simulink model "BIKENON"  (R2023a)
settings: Solver=ode113  StartTime=0.0  StopTime=15  MaxStep=1  RelTol=1e-3  AbsTol=1e-3
values from neighbouring files (symbols this model uses):
  u0 = initial_velocities(v_idx)    [perform_simulations.m]    (also in plots.m = initialVelocities(vIdx))
undefined symbols (not defined in the file or in its folder): a, b, Cf, Cr, G, I, M, r0, v0
settings Model: Creator=pisup  LastModifiedBy=kvadner
settings SolverCC: AutoScaleAbsTol=off  AlgebraicLoopSolver=TrustRegion
settings DataIOCC: SaveFormat=Array  SignalLoggingSaveFormat=ModelDataLogs  SaveOutput=off  SaveTime=off  ReturnWorkspaceOutputs=off
settings OptimizationCC: BlockReduction=off  BooleanDataType=off  ExpressionDepthLimit=2147483647  InitFltsAndDblsToZero=on  LifeSpan=inf
settings DebuggingCC: SaveWithParameterizedLinksMsg=none  UnderspecifiedInitializationDetection=Classic  MergeDetectMultiDrivingBlocksExec=none  SignalResolutionControl=TryResolveAllWithWarning  MultiTaskDSMMsg=warning  MultiTaskCondExecSysMsg=none  FcnCallInpInsideContextMsg=warning  UnconnectedInputMsg=warning  UnconnectedOutputMsg=warning  UnconnectedLineMsg=warning  StateNameClashWarn=warning  SFUnexpectedBacktrackingDiag=warning  SFNoUnconditionalDefaultTransitionDiag=warning  SFExecutionAtInitializationDiag=none  ArithmeticOperatorsInVariantConditions=warning
settings HardwareCC: ProdBitPerPointer=32  ProdBitPerSizeT=32  ProdBitPerPtrDiffT=32  ProdLargestAtomicFloat=None  ProdIntDivRoundTo=Undefined  ProdEndianess=Unspecified  ProdWordSize=32  ProdHWDeviceType=32-bit Generic  TargetUnknown=on
settings ModelReferenceCC: EnableRefExpFcnMdlSchedulingChecks=on  PropagateSignalLabelsOutOfModel=off
settings RTWCC: TemplateMakefile=grt_vc.tmf
settings CodeAppCC: StateflowObjectComments=on
settings GRTTargetCC: TargetLangStandard=C89/C90 (ANSI)  CombineOutputUpdateFcns=off  GRTInterface=on
settings ConfigComp: CovMetricSettings=dw  CovSaveCumulativeToWorkspaceVar=on  CovSaveSingleToWorkspaceVar=on

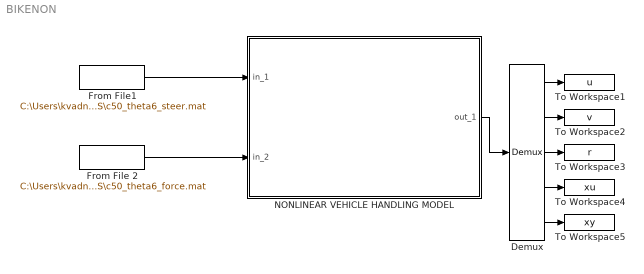
== system BIKENON ==
  Demux : Demux  Outputs=5
      settings: DisplayOption=none
  From File 2 : FromFile  FileName=C:\Users\kvadner\Desktop\Research\Fault Detection Markov MDP\Simulink\Files for HW2\Input Maneuvers\SRS\c50_theta6_force.mat  SampleTime=0
  From File1 : FromFile  FileName=C:\Users\kvadner\Desktop\Research\Fault Detection Markov MDP\Simulink\Files for HW2\Input Maneuvers\SRS\c50_theta6_steer.mat  SampleTime=0
  NONLINEAR VEHICLE HANDLING MODEL : Subsystem
  To Workspace1 : ToWorkspace  VariableName=u
      settings: MaxDataPoints=10000
  To Workspace2 : ToWorkspace  VariableName=v
      settings: MaxDataPoints=10000
  To Workspace3 : ToWorkspace  VariableName=r
      settings: MaxDataPoints=10000
  To Workspace4 : ToWorkspace  VariableName=xu
      settings: MaxDataPoints=10000
  To Workspace5 : ToWorkspace  VariableName=xy
      settings: MaxDataPoints=10000
  wires:
  Demux/3 -> To Workspace3/1
  Demux/2 -> To Workspace2/1
  Demux/1 -> To Workspace1/1
  NONLINEAR VEHICLE HANDLING MODEL/1(out_1) -> Demux/1
  Demux/4 -> To Workspace4/1
  Demux/5 -> To Workspace5/1
  From File1/1 -> NONLINEAR VEHICLE HANDLING MODEL/1(in_1)
  From File 2/1 -> NONLINEAR VEHICLE HANDLING MODEL/2(in_2)

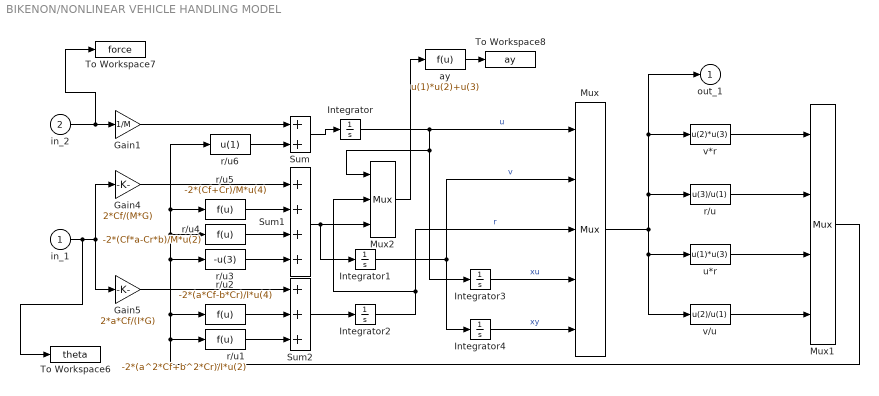
== system BIKENON/NONLINEAR VEHICLE HANDLING MODEL ==
  in_1 : Inport
  in_2 : Inport  Port=2
  Gain1 : Gain  Gain=1/M  SaturateOnIntegerOverflow=on  OutDataTypeStr=Inherit: Same as input  ParamDataTypeStr=Inherit: Same as input
  Gain4 : Gain  Gain=2*Cf/(M*G)  SaturateOnIntegerOverflow=on  OutDataTypeStr=Inherit: Same as input  ParamDataTypeStr=Inherit: Same as input
  Gain5 : Gain  Gain=2*a*Cf/(I*G)  SaturateOnIntegerOverflow=on  OutDataTypeStr=Inherit: Same as input  ParamDataTypeStr=Inherit: Same as input
  Integrator : Integrator  InitialCondition=u0
  Integrator1 : Integrator  InitialCondition=v0
  Integrator2 : Integrator  InitialCondition=r0
  Integrator3 : Integrator
  Integrator4 : Integrator
  Mux : Mux  Inputs=5
  Mux1 : Mux
  Mux2 : Mux  Inputs=3
  Sum : Sum  InputSameDT=on  SaturateOnIntegerOverflow=on  OutDataTypeStr=Inherit: Same as first input
  Sum1 : Sum  Inputs=++++  InputSameDT=on  SaturateOnIntegerOverflow=on  OutDataTypeStr=Inherit: Same as first input
  Sum2 : Sum  Inputs=+++  InputSameDT=on  SaturateOnIntegerOverflow=on  OutDataTypeStr=Inherit: Same as first input
  To Workspace6 : ToWorkspace  VariableName=theta
      settings: MaxDataPoints=10000
  To Workspace7 : ToWorkspace  VariableName=force
      settings: MaxDataPoints=10000
  To Workspace8 : ToWorkspace  VariableName=ay
      settings: MaxDataPoints=10000
  ay : Fcn  Expr=u(1)*u(2)+u(3)
  r/u : Fcn  Expr=u(3)/u(1)
  r/u1 : Fcn  Expr=-2*(a^2*Cf+b^2*Cr)/I*u(2)
  r/u2 : Fcn  Expr=-2*(a*Cf-b*Cr)/I*u(4)
  r/u3 : Fcn  Expr=-u(3)
  r/u4 : Fcn  Expr=-2*(Cf*a-Cr*b)/M*u(2)
  r/u5 : Fcn  Expr=-2*(Cf+Cr)/M*u(4)
  r/u6 : Fcn  Expr=u(1)
  u*r : Fcn  Expr=u(1)*u(3)
  v*r : Fcn  Expr=u(2)*u(3)
  v/u : Fcn  Expr=u(2)/u(1)
  out_1 : Outport  InitialOutput=0
  wires:
  Sum/1 -> Integrator/1
  Integrator/1 -> Mux/1, Integrator3/1, Mux2/1  "u"
  Integrator1/1 -> Mux/2, Integrator4/1  "v"
  Integrator2/1 -> Mux/3, Mux2/2  "r"
  Sum1/1 -> Mux2/3, Integrator1/1
  Sum2/1 -> Integrator2/1
  v*r/1 -> Mux1/1
  r/u/1 -> Mux1/2
  u*r/1 -> Mux1/3
  v/u/1 -> Mux1/4
  Mux/1 -> v/u/1, u*r/1, out_1/1, v*r/1, r/u/1
  in_1/1 -> To Workspace6/1, Gain4/1, Gain5/1
  r/u1/1 -> Sum2/3
  r/u2/1 -> Sum2/2
  r/u6/1 -> Sum/2
  r/u3/1 -> Sum1/4
  r/u4/1 -> Sum1/3
  r/u5/1 -> Sum1/2
  Gain5/1 -> Sum2/1
  Gain4/1 -> Sum1/1
  Mux1/1 -> r/u1/1, r/u2/1, r/u3/1, r/u4/1, r/u5/1, r/u6/1
  Gain1/1 -> Sum/1
  in_2/1 -> To Workspace7/1, Gain1/1
  Integrator3/1 -> Mux/4  "xu"
  Integrator4/1 -> Mux/5  "xy"
  Mux2/1 -> ay/1
  ay/1 -> To Workspace8/1
